simulink model "ASK"  (Simulink 8.2)
settings: Solver=ode45  StartTime=0.0  StopTime=10.0  RelTol=1e-3
libraries: dsparch4 x3, commsink2 x2, commchan3 x1, commrandsrc2 x1, dspsigops x1
settings Model: Creator=Yi_Liu  LastModifiedBy=Yi_Liu
settings DataIOCC: SignalLoggingSaveFormat=Dataset
settings OptimizationCC: ExpressionDepthLimit=128
settings DebuggingCC: FcnCallInpInsideContextMsg=EnableAllAsError  StateNameClashWarn=none
settings GRTTargetCC: CombineOutputUpdateFcns=on  GRTInterface=off

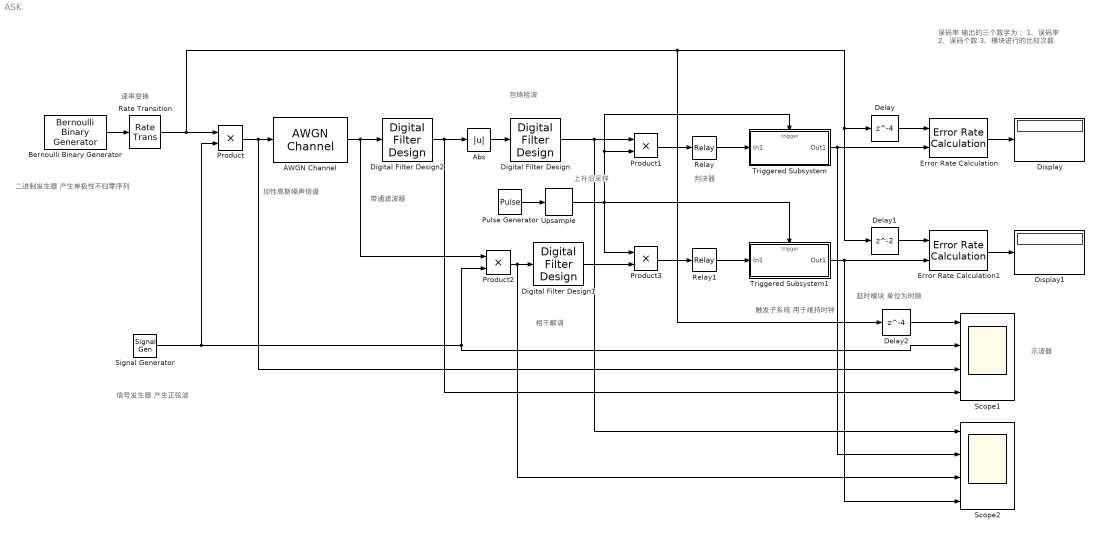
== system ASK ==
  note: 相干解调
  note: 包络检波
  note: 误码率
      | 输出的三个数字为：
      | 1、误码率
      | 2、误码个数
      | 3、模块进行的比较次数
  note: 延时模块 单位为时隙
  note: 示波器
  note: 触发子系统
      | 用于维持时钟
  note: 判决器
  note: 上升沿采样
  note: 带通滤波器
  note: 加性高斯噪声信道
  note: 信号发生器
      | 产生正弦波
  note: 速率变换
  note: 二进制发生器
      | 产生单极性不归零序列
  AWGN Channel : commchan3/AWGN Channel  InputProcessing=Columns as channels (frame based)  seed=61  noiseMode=Variance from mask  EbNodB=10  EsNodB=10  SNRdB=15  bitsPerSym=1  Ps=1  Tsym=1  variance=0.05
  Abs : Abs
  Bernoulli Binary Generator : commrandsrc2/Bernoulli Binary Generator  P=0.5  seed=61  Ts=1/500  frameBased=off  sampPerFrame=1  orient=off  outDataType=double
  Delay : Delay  DelayLength=4  InitialCondition=0  SampleTime=0.0001
  Delay1 : Delay  InitialCondition=0  SampleTime=0.0001
  Delay2 : Delay  DelayLength=4  InitialCondition=0  SampleTime=0.0001
  Digital Filter Design : dsparch4/Digital Filter Design  mwdsp_browser_bugfix_var=off
  Digital Filter Design1 : dsparch4/Digital Filter Design  mwdsp_browser_bugfix_var=off
  Digital Filter Design2 : dsparch4/Digital Filter Design  mwdsp_browser_bugfix_var=off
  Display : Display
  Display1 : Display
  Error Rate Calculation : commsink2/Error Rate Calculation  N=0  st_delay=0  cp_mode=Entire frame  subframe=[]  PMode=Port  WsName=ErrorVec  RsMode2=off  stop=off  numErr=100  maxBits=1e6
  Error Rate Calculation1 : commsink2/Error Rate Calculation  N=0  st_delay=0  cp_mode=Entire frame  subframe=[]  PMode=Port  WsName=ErrorVec  RsMode2=off  stop=off  numErr=100  maxBits=1e6
  Product{,1..3} (4 alike) : Product
  Pulse Generator : DiscretePulseGenerator  Period=10  PulseWidth=5  SampleTime=1/10000
  Rate Transition : RateTransition  OutPortSampleTime=1/10000
  Relay : Relay  OnSwitchValue=0.28  OffSwitchValue=0.28  SampleTime=0.0001
  Relay1 : Relay  OnSwitchValue=0.12  OffSwitchValue=0.12  SampleTime=0.00002
  Scope1 : Scope  NumInputPorts=4
      settings: YMin=-2~-5~-2~-2  YMax=2~5~2~2
  Scope2 : Scope  NumInputPorts=4
      settings: YMin=-2~-2~-2~-2  YMax=2~2~2~2  SaveName=ScopeData2
  Signal Generator : SignalGenerator  Frequency=2*pi*1000  Units=rad/sec
  Triggered Subsystem : Subsystem  TreatAsAtomicUnit=on
  Triggered Subsystem1 : Subsystem  TreatAsAtomicUnit=on
  Upsample : dspsigops/Upsample  N=10  phase=0  RateOptions=Allow multirate processing  ic=0  mode=Unused parameter value
  wires:
  Pulse Generator/1 -> Upsample/1
  Error Rate Calculation/1 -> Display/1
  Bernoulli Binary Generator/1 -> Rate Transition/1
  Abs/1 -> Digital Filter Design/1
  Digital Filter Design/1 -> Scope2/1, Product1/1
  Upsample/1 -> Triggered Subsystem/Trigger, Product1/2, Triggered Subsystem1/Trigger, Product3/1
  Product2/1 -> Scope2/3, Digital Filter Design1/1
  Digital Filter Design1/1 -> Product3/2
  Product3/1 -> Relay1/1
  Product1/1 -> Relay/1
  Error Rate Calculation1/1 -> Display1/1
  Triggered Subsystem1/1(Out1) -> Scope2/4, Error Rate Calculation1/2
  Relay1/1 -> Triggered Subsystem1/1(In1)
  Relay/1 -> Triggered Subsystem/1(In1)
  Triggered Subsystem/1(Out1) -> Scope2/2, Error Rate Calculation/2
  AWGN Channel/1 -> Product2/1, Digital Filter Design2/1
  Delay/1 -> Error Rate Calculation/1
  Rate Transition/1 -> Delay2/1, Delay1/1, Delay/1, Product/1
  Delay2/1 -> Scope1/1
  Delay1/1 -> Error Rate Calculation1/1
  Product/1 -> Scope1/3, AWGN Channel/1
  Signal Generator/1 -> Scope1/2, Product2/2, Product/2
  Digital Filter Design2/1 -> Scope1/4, Abs/1

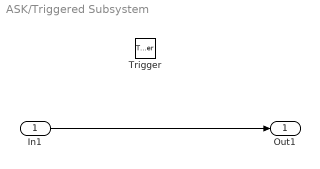
== system ASK/Triggered Subsystem ==
  In1 : Inport
  Trigger : TriggerPort
  Out1 : Outport
  wires:
  In1/1 -> Out1/1

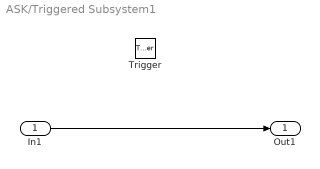
== system ASK/Triggered Subsystem1 ==
  In1 : Inport
  Trigger : TriggerPort
  Out1 : Outport
  wires:
  In1/1 -> Out1/1
